simulink model "prob2"  (R2020b)
settings: Solver=FixedStepAuto  StartTime=0.0  StopTime=10.0  RelTol=1e-3
model workspace (MAT data in the model file):
  b = 1
  k1 = 0.1
  k2 = 0.01
  m1 = 100
  m2 = 200
settings Model: Creator=AVM  LastModifiedBy=AVM

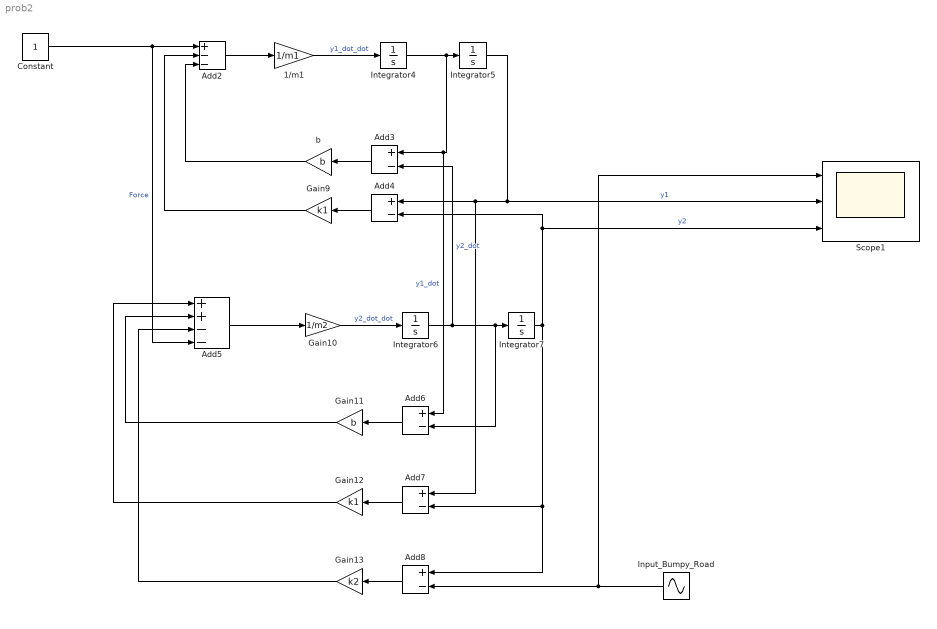
== system prob2 ==
  1/m1 : Gain  Gain=1/m1
  Add2 : Sum  Inputs=+--
  Add{3..4,6..8} (5 alike) : Sum  Inputs=+-
  Add5 : Sum  Inputs=++--
  Constant : Constant
  Gain10 : Gain  Gain=1/m2
  Gain11 : Gain  Gain=b
  Gain12 : Gain  Gain=k1
  Gain13 : Gain  Gain=k2
  Gain9 : Gain  Gain=k1
  Input_Bumpy_Road : Sin  SampleTime=0
  Integrator{4..7} (4 alike) : Integrator
  Scope1 : Scope  NumInputPorts=3
  b : Gain  Gain=b
  wires:
  Add7/1 -> Gain12/1
  Gain13/1 -> Add5/3
  Add8/1 -> Gain13/1
  Input_Bumpy_Road/1 -> Scope1/1, Add8/2
  Add4/1 -> Gain9/1
  Constant/1 -> Add5/4, Add2/1  "Force"
  Gain10/1 -> Integrator6/1  "y2_dot_dot"
  Gain12/1 -> Add5/1
  Add6/1 -> Gain11/1
  Integrator7/1 -> Add4/2, Scope1/3, Add8/1, Add7/2  "y2"
  Gain9/1 -> Add2/2
  Integrator5/1 -> Scope1/2, Add7/1, Add4/1  "y1"
  Integrator4/1 -> Integrator5/1, Add6/1, Add3/1  "y1_dot"
  Integrator6/1 -> Add3/2, Add6/2, Integrator7/1  "y2_dot"
  Add5/1 -> Gain10/1
  Add3/1 -> b/1
  b/1 -> Add2/3
  1/m1/1 -> Integrator4/1  "y1_dot_dot"
  Gain11/1 -> Add5/2
  Add2/1 -> 1/m1/1
